simulink model "P_3_1_h_Predacio_modell"  (R2021b)
settings: Solver=ode4  StartTime=0.0  StopTime=100  FixedStep=1  RelTol=1e-3
settings Model: Creator=davidpaksi  LastModifiedBy=davidpaksi

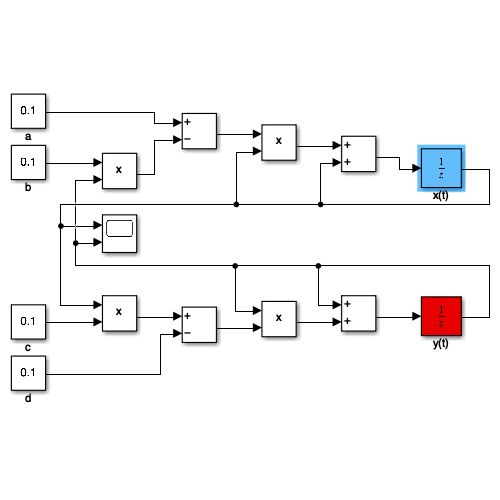
[thumbnail: Simulink's stored preview of the top-level diagram]
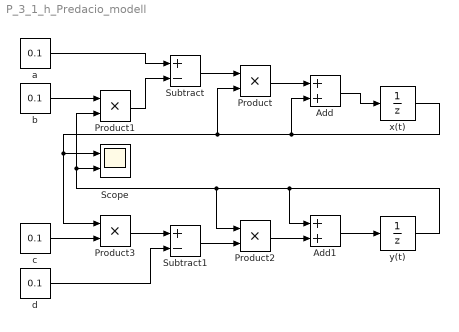
== system P_3_1_h_Predacio_modell ==
  Add : Sum
  Add1 : Sum
  Product{,1..3} (4 alike) : Product
  Scope : Scope  NumInputPorts=2
  Subtract : Sum  Inputs=+-
  Subtract1 : Sum  Inputs=+-
  a : Constant  Value=0.1
  b : Constant  Value=0.1
  c : Constant  Value=0.1
  d : Constant  Value=0.1
  x(t) : UnitDelay  InitialCondition=1  HasFrameUpgradeWarning=on
  y(t) : UnitDelay  InitialCondition=2  HasFrameUpgradeWarning=on
  wires:
  Add/1 -> x(t)/1
  x(t)/1 -> Add/2, Product/2, Scope/1, Product3/1
  a/1 -> Subtract/1
  Product1/1 -> Subtract/2
  b/1 -> Product1/1
  y(t)/1 -> Product2/1, Scope/2, Product1/2, Add1/1
  Add1/1 -> y(t)/1
  Product2/1 -> Add1/2
  Subtract1/1 -> Product2/2
  c/1 -> Product3/2
  Product/1 -> Add/1
  Subtract/1 -> Product/1
  Product3/1 -> Subtract1/1
  d/1 -> Subtract1/2
